simulink model "matrix_mult_cosim"  (R2017a)
settings: Solver=VariableStepAuto  StartTime=0.0  StopTime=29  RelTol=1e-3
undefined symbols (not defined in the file or in its folder): A, N
libraries: xbsIndex_r4 x129, JTAGRuntimeCosim_r4 x1
(part 2 of 2)

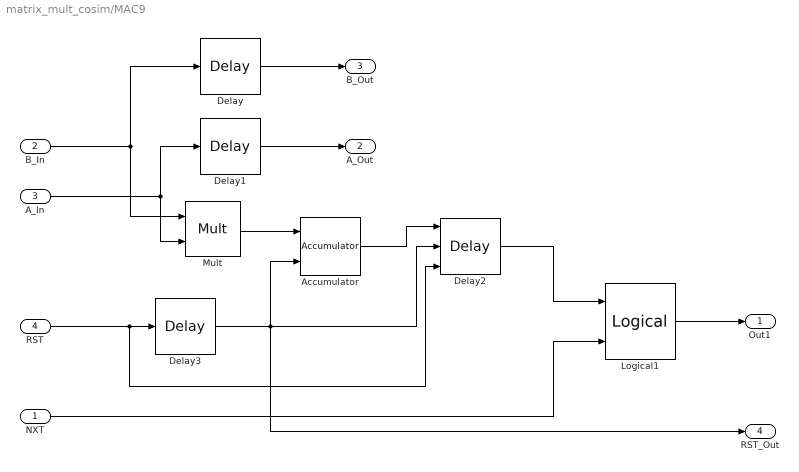
== system matrix_mult_cosim/MAC9 ==
  NXT : Inport
  B_In : Inport  Port=2
  A_In : Inport  Port=3
  RST : Inport  Port=4
  Accumulator : xbsIndex_r4/Accumulator  operation=Add  n_bits=16  overflow=Wrap  scale=1  rst=on  hasbypass=off  infoeditControl=reset for floating point data type must be asserted for a minimum of 2 cycles  en=off  latency=1  msb_inp=100  msb=100  lsb=-100  use_behavioral_HDL=on  implementation=Fabric  dbl_ovrd=off  block_type=accum
  Delay : xbsIndex_r4/Delay  rst=off  infoeditControl=Selection of Reset will increase slice count due to use of real FFs and instead of SRLs  en=off  latency=1  reg_retiming=off  dbl_ovrd=off  block_type=delay
  Delay1 : xbsIndex_r4/Delay  rst=off  infoeditControl=Selection of Reset will increase slice count due to use of real FFs and instead of SRLs  en=off  latency=1  reg_retiming=off  dbl_ovrd=off  block_type=delay
  Delay2 : xbsIndex_r4/Delay  rst=on  infoeditControl=Selection of Reset will increase slice count due to use of real FFs and instead of SRLs  en=on  latency=1  reg_retiming=off  dbl_ovrd=off  block_type=delay
  Delay3 : xbsIndex_r4/Delay  rst=off  infoeditControl=Selection of Reset will increase slice count due to use of real FFs and instead of SRLs  en=off  latency=1  reg_retiming=off  dbl_ovrd=off  block_type=delay
  Logical1 : xbsIndex_r4/Logical  logical_function=OR  inputs=2  en=off  latency=0  precision=Full  arith_type=Unsigned  n_bits=16  bin_pt=0  align_bp=on  dbl_ovrd=off  block_type=logical
  Mult : xbsIndex_r4/Mult  precision=User Defined  arith_type="Signed  (2's comp)"  n_bits=16  bin_pt=0  quantization=Truncate  overflow=Wrap  en=off  latency=3  use_behavioral_HDL=off  opt=Speed  use_embedded=on  optimum_pipeline=off  pipeline=on  dbl_ovrd=off  use_rpm=on  placement_style=Triangular  block_type=mult
  Out1 : Outport
  A_Out : Outport  Port=2
  B_Out : Outport  Port=3
  RST_Out : Outport  Port=4
  wires:
  RST/1 -> Delay2/3, Delay3/1
  Mult/1 -> Accumulator/1
  B_In/1 -> Delay/1, Mult/1
  A_In/1 -> Delay1/1, Mult/2
  Delay/1 -> B_Out/1
  Delay1/1 -> A_Out/1
  Accumulator/1 -> Delay2/1
  Logical1/1 -> Out1/1
  Delay3/1 -> Accumulator/2, Delay2/2, RST_Out/1
  Delay2/1 -> Logical1/1
  NXT/1 -> Logical1/2
